simulink subsystem "MPC_control"  (R2024a)
settings: Solver=VariableStepAuto  StartTime=0.0  StopTime=10.0  RelTol=1e-3
libraries: mpclib x1
settings Model: Creator=Peter  LastModifiedBy=Peter

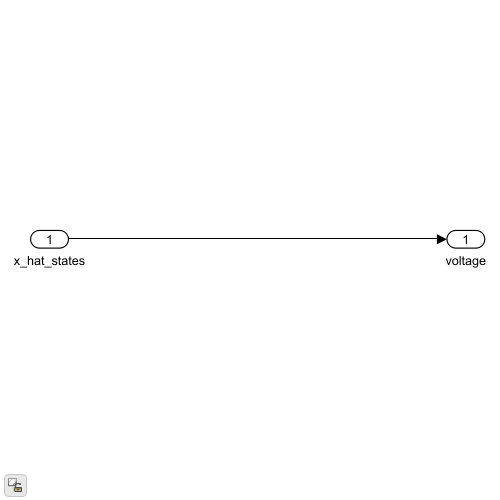
[thumbnail: Simulink's stored preview of the top-level diagram]
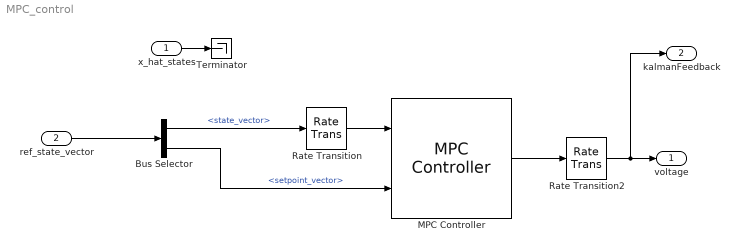
== system MPC_control ==
  x_hat_states : Inport
  ref_state_vector : Inport  Port=2
  Bus Selector : BusSelector  OutputSignals=state_vector,setpoint_vector
  MPC Controller : mpclib/MPC Controller  SCDEnableBlockLinearizationSpecification=on  mpcobj=mpc1  is_multiple=0  enable_value=0  return_u0=off  updateMPCinCallerWorkspace=on  md_inport=off  mv_inport=off  uref_inport=off  return_cost=off  return_mvseq=off  return_qpstatus=off  return_xseq=off  return_state=off  return_ovseq=off  state_inport=off  umin_inport=off  umax_inport=off  ymin_inport=off  ymax_inport=off  cc_inport=off  ywt_inport=off  uwt_inport=off  duwt_inport=off  rhoeps_inport=off  pm_inport=off  MaximumP=10  HorizonChoice=FixedHorizon  n_ts=0.02  n_p=10  n_mv=1  n_md=0  n_ud=0  n_mo=6  n_uo=0  BlockDataType=single  SampleTimeInherited=off  switch_inport=off
  Rate Transition : RateTransition
  Rate Transition2 : RateTransition
  Terminator : Terminator
  voltage : Outport
  kalmanFeedback : Outport  Port=2  OutDataTypeStr=single
  wires:
  MPC Controller/1 -> Rate Transition2/1
  ref_state_vector/1 -> Bus Selector/1
  Rate Transition/1 -> MPC Controller/1
  x_hat_states/1 -> Terminator/1
  Bus Selector/1 -> Rate Transition/1  "<state_vector>"
  Rate Transition2/1 -> voltage/1, kalmanFeedback/1
  Bus Selector/2 -> MPC Controller/2  "<setpoint_vector>"
